simulink model "LVLineal"  (R2020b)
settings: Solver=FixedStepAuto  StartTime=0.0  StopTime=10  FixedStep=0.01  MaxStep=0.01  RelTol=1e-3
values from neighbouring files (symbols this model uses):
  a = pred(1)    [Curva_linealidad.m]    (also in FindEquations.m; Linealizar.m; yue_bifur.m = linspace(a0,a1,N))
  alpha = cap(1)    [Curva_linealidad.m]    (also in FindEquations.m; Linealizar.m)
  b = pred(2)    [Curva_linealidad.m]    (also in FindEquations.m; Linealizar.m)
  beta = cap(2)    [Curva_linealidad.m]    (also in FindEquations.m; Linealizar.m)
  c = pred(3)    [Curva_linealidad.m]    (also in FindEquations.m; Linealizar.m)
  chi = cap(3)    [Curva_linealidad.m]    (also in FindEquations.m; Linealizar.m)
  K = cap(4)    [Curva_linealidad.m]    (also in FindEquations.m; Linealizar.m; Untitled.m = num2str(cap(4)))
  r1 = rep(1)    [Curva_linealidad.m]    (also in FindEquations.m; Linealizar.m)
  r2 = rep(2)    [Curva_linealidad.m]    (also in FindEquations.m; Linealizar.m)
  r3 = rep(3)    [Curva_linealidad.m]    (also in FindEquations.m; Linealizar.m)
  u0 = ui(1)    [Linealizar.m]
  U1 = entradas(i)    [Curva_linealidad.m]    (also in FindEquations.m = ui(1); Horario.m = 10; Linealizar.m = ui(1) + delta; Untitled.m = 0)
  x10 = 2000    [Curva_linealidad.m]    (also in Linealizar.m = xe(1))
  x20 = 175    [Curva_linealidad.m]    (also in Linealizar.m = xe(2))
  x30 = 200    [Curva_linealidad.m]    (also in Linealizar.m = xe(3))
settings Model: Creator=mluser  LastModifiedBy=sofia
settings DataIOCC: SaveOutput=off  SignalLogging=off  DSMLogging=off  SaveTime=off  ReturnWorkspaceOutputs=off
settings DebuggingCC: SFMachineParentedDataDiag=error

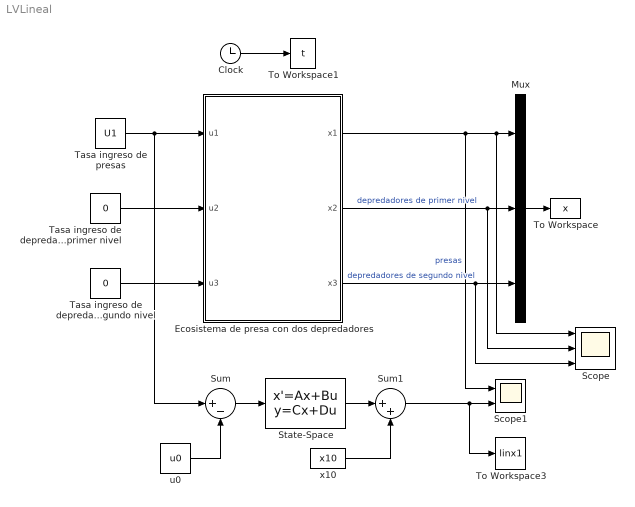
== system LVLineal ==
  Clock : Clock
  Ecosistema de presa con dos depredadores : Subsystem  mask(Extensión del modelo Lotka-Volterra para un ecosistema depredador/depredador/presa){ci=[x10 x20 x30], ri=[r1 r2 r3], K=K, ic=[a b c], pc=[alpha beta chi]}
      mask prompts: ci "Poblaciones iniciales [x10 x20 x30]"; ri "Tasas de crecimiento intrínseco  [r1 r2 r3]"; K "Capacidad de carga de las presas (K)"; ic "Constantes de interacción [a b c]"; pc "Constantes de proporcionalidad para la capacidad de carga [alpha beta chi]"
      mask help: Sistema de tres ecuaciones diferenciales de primer orden no lineales que describen el comportamiento de un sistema ecológico de tres niveles tróficos: población presa (nivel trófico 1, es depredada por todos), población de depredador de primer nivel (nivel trófico 2, es depredador de la población presa pero también es presa del depredador de segundo nivel) y población de depredador de segundo nivel (nivel trófico 3, es depredador de todos).
      mask init:
      | r1 = ri(1);
      | r2 = ri(2);
      | r3 = ri(3);
      | 
      | 
      | a = ic(1);
      | b = ic(2);
      | c = ic(3);
      | 
      | alpha = pc(1);
      | beta = pc(2);
      | chi = pc(3);
      | 
      | x10 = ci(1);
      | x20 = ci(2);
      | x30 = ci(3);
  Mux : Mux  Inputs=3
  Scope : Scope  NumInputPorts=3
  Scope1 : Scope  NumInputPorts=2
  State-Space : StateSpace  A=[-0.2605 -15.8113 0; 0.1816 -1.1129 -3.8712;0 0.0620 -0.62]  B=[1;0;0]  C=[1 0 0]  D=0  InitialCondition=0
  Sum : Sum  Inputs=|+-
  Sum1 : Sum  Inputs=|++
  Tasa ingreso de depredadores de primer nivel : Constant  Value=0
  Tasa ingreso de depredadores de segundo nivel : Constant  Value=0
  Tasa ingreso de presas : Constant  Value=U1
  To Workspace : ToWorkspace  VariableName=x  SampleTime=-1
  To Workspace1 : ToWorkspace  VariableName=t  SampleTime=-1
  To Workspace3 : ToWorkspace  VariableName=linx1  SampleTime=-1
  u0 : Constant  Value=u0
  x10 : Constant  Value=x10
  wires:
  Tasa ingreso de presas/1 -> Sum/1, Ecosistema de presa con dos depredadores/1(u1)
  Tasa ingreso de depredadores de segundo nivel/1 -> Ecosistema de presa con dos depredadores/3(u3)
  Tasa ingreso de depredadores de primer nivel/1 -> Ecosistema de presa con dos depredadores/2(u2)
  Ecosistema de presa con dos depredadores/1("x1 ") -> Scope1/1, Scope/1, Mux/1  "presas"
  Ecosistema de presa con dos depredadores/2("x2 ") -> Scope/2, Mux/2  "depredadores de primer nivel"
  Ecosistema de presa con dos depredadores/3("x3 ") -> Scope/3, Mux/3  "depredadores de segundo nivel"
  Mux/1 -> To Workspace/1
  Clock/1 -> To Workspace1/1
  Sum/1 -> State-Space/1
  u0/1 -> Sum/2
  State-Space/1 -> Sum1/1
  x10/1 -> Sum1/2
  Sum1/1 -> To Workspace3/1, Scope1/2

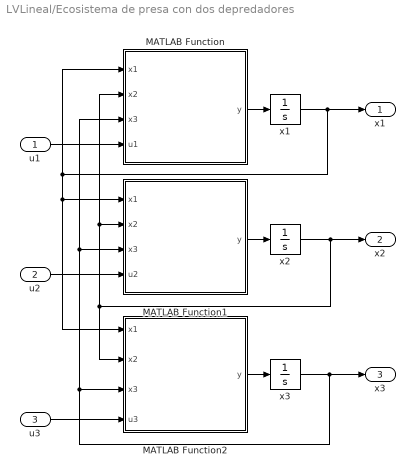
== system LVLineal/Ecosistema de presa con dos depredadores ==
  u1 : Inport
  u2 : Inport  Port=2
  u3 : Inport  Port=3
  MATLAB Function : MATLAB Function  TreatAsAtomicUnit=on
  MATLAB Function1 : MATLAB Function  TreatAsAtomicUnit=on
  MATLAB Function2 : MATLAB Function  TreatAsAtomicUnit=on
  x1 : Integrator  InitialCondition=x10  LimitOutput=on  LowerSaturationLimit=0
  x2 : Integrator  InitialCondition=x20  LimitOutput=on  LowerSaturationLimit=0
  x3 : Integrator  InitialCondition=x30  LimitOutput=on  LowerSaturationLimit=0
  "x1 " : Outport
  "x2 " : Outport  Port=2
  "x3 " : Outport  Port=3
  wires:
  x1/1 -> "x1 "/1, MATLAB Function/1(x1), MATLAB Function2/1(x1), MATLAB Function1/1(x1)
  MATLAB Function1/1(y) -> x2/1
  u1/1 -> MATLAB Function/4(u1)
  x3/1 -> "x3 "/1, MATLAB Function1/3(x3), MATLAB Function/3(x3), MATLAB Function2/3(x3)
  MATLAB Function2/1(y) -> x3/1
  x2/1 -> "x2 "/1, MATLAB Function/2(x2), MATLAB Function1/2(x2), MATLAB Function2/2(x2)
  MATLAB Function/1(y) -> x1/1
  u2/1 -> MATLAB Function1/4(u2)
  u3/1 -> MATLAB Function2/4(u3)

== matlab function LVLineal/Ecosistema de presa con dos depredadores/MATLAB Function ==
  data: r1 parameter; a parameter; b parameter; K parameter; y output; x1 input; x2 input; x3 input; u1 input
function y = fcn(r1,a,b,K,x1,x2,x3,u1)
y = r1*x1*(1-(x1/K))-a*x1*x2-b*x1*x3 + u1;

== matlab function LVLineal/Ecosistema de presa con dos depredadores/MATLAB Function1 ==
  data: r2 parameter; alpha parameter; c parameter; y output; x1 input; x2 input; x3 input; u2 input
function y = fcn(r2,alpha,c,x1,x2,x3,u2)
    term=0;
    if alpha ~=0
        term = (x2/(alpha*x1));
        y = r2*x2*(1-term)-c*x2*x3+u2;
    else
        y = 0;
    end
end

== matlab function LVLineal/Ecosistema de presa con dos depredadores/MATLAB Function2 ==
  data: r3 parameter; beta parameter; chi parameter; x1 input; x2 input; x3 input; y output; u3 input
function y = fcn(r3,beta,chi,x1,x2,x3,u3)
    term = 0;
    if not(beta == 0 && chi == 0)
        term = (x3/(beta*x1+chi*x2));
        y = r3*x3*(1-term)+u3;
    else
        y = 0;
    end
end
